simulink model "consumocalcio"  (Simulink 7.5)
settings: Solver=ode45  StartTime=0.0  StopTime=10.0  RelTol=1e-3
settings Model: Creator=My Laptop  LastModifiedBy=My Laptop

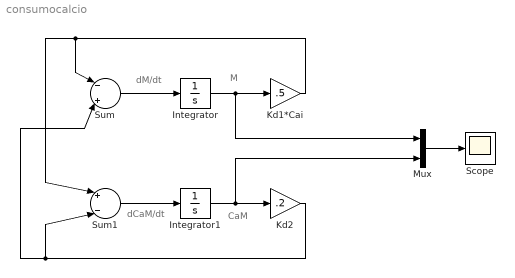
== system consumocalcio ==
  note: M
  note: CaM
  note: dM/dt
  note: dCaM/dt
  Integrator : Integrator  InitialCondition=5
  Integrator1 : Integrator  InitialCondition=7
  Kd1*Cai : Gain  Gain=.5  ParameterDataType=fixdt(1, 16)  ParameterScaling=2^0  OutDataType=fixdt(1, 16)  OutScaling=2^0
  Kd2 : Gain  Gain=.2  ParameterDataType=fixdt(1, 16)  ParameterScaling=2^0  OutDataType=fixdt(1, 16)  OutScaling=2^0
  Mux : Mux  Inputs=2
  Scope : Scope
  Sum : Sum  Inputs=|-|+|  OutDataType=fixdt(1, 16)  OutScaling=2^0
  Sum1 : Sum  Inputs=|+|-|  OutDataType=fixdt(1, 16)  OutScaling=2^0
  wires:
  Mux/1 -> Scope/1
  Integrator1/1 -> Kd2/1, Mux/2
  Integrator/1 -> Kd1*Cai/1, Mux/1
  Kd1*Cai/1 -> Sum/1, Sum1/1
  Sum1/1 -> Integrator1/1
  Sum/1 -> Integrator/1
  Kd2/1 -> Sum/2, Sum1/2
